simulink model "MIMOforRRR"  (R2019b)
settings: Solver=ode3  StartTime=0.0  StopTime=10.0  RelTol=1e-3
libraries: roblocks x3
settings Model: Creator=mads  LastModifiedBy=mads

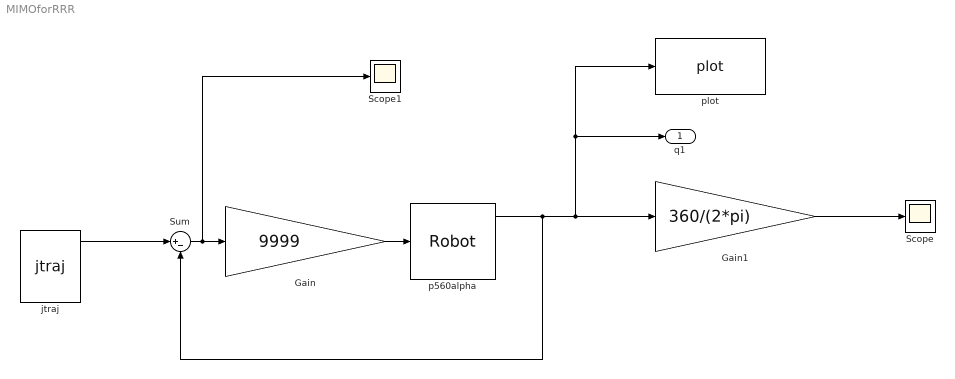
== system MIMOforRRR ==
  Gain : Gain  Gain=9999
  Gain1 : Gain  Gain=360/(2*pi)
  Scope : Scope
  Scope1 : Scope
  Sum : Sum  Inputs=|+-
  jtraj : roblocks/Toolbox/jtraj  q0=[0 0 0]  qf=[pi/2 -pi/4 -pi/4]  tmax=2  ts=0.02
  p560alpha : roblocks/Arm/Robot  robot=p560alpha  q0=[0 0 0]
  plot : roblocks/Arm/plot  robot=p560alpha  fps=5  holdplot=on
  q1 : Outport  VectorParamsAs1DForOutWhenUnconnected=off
  wires:
  jtraj/1 -> Sum/1
  Sum/1 -> Scope1/1, Gain/1
  Gain/1 -> p560alpha/1
  p560alpha/1 -> q1/1, plot/1, Gain1/1, Sum/2
  Gain1/1 -> Scope/1
